simulink model "SimulationOfFuruta"  (R2017a)
settings: Solver=ode4  StartTime=0.0  StopTime=20  RelTol=1e-3  EnableMultiTasking=on
settings Model: Creator=marce  LastModifiedBy=felip
settings DataIOCC: LimitDataPoints=on  SaveFormat=Array
settings OptimizationCC: LifeSpan=inf
settings DebuggingCC: SFUnexpectedBacktrackingDiag=warning  SFNoUnconditionalDefaultTransitionDiag=warning  SFExecutionAtInitializationDiag=none
settings HardwareCC: ProdBitPerPointer=32  ProdBitPerSizeT=32  ProdBitPerPtrDiffT=32  ProdLargestAtomicFloat=None  ProdIntDivRoundTo=Undefined  ProdEndianess=Unspecified  ProdWordSize=32  ProdHWDeviceType=32-bit Generic
settings ModelReferenceCC: PropagateSignalLabelsOutOfModel=off
settings GRTTargetCC: TargetLangStandard=C89/C90 (ANSI)  GeneratePreprocessorConditionals=Disable all
settings ConfigComp: CovMetricSettings=dw  CovHtmlReporting=on  CovSaveCumulativeToWorkspaceVar=on  CovSaveSingleToWorkspaceVar=on  CovExternalEMLEnable=off

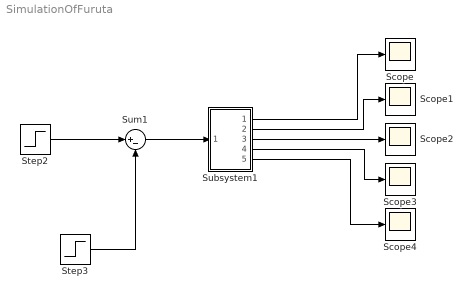
== system SimulationOfFuruta ==
  Scope{,1..4} (5 alike) : Scope
  Step2 : Step  SampleTime=0
  Step3 : Step  SampleTime=0
  Subsystem1 : Subsystem
  Sum1 : Sum  Inputs=|+-
  wires:
  Subsystem1/4(Out4) -> Scope3/1
  Subsystem1/3(Out3) -> Scope2/1
  Subsystem1/5(Out5) -> Scope4/1
  Subsystem1/2(Out2) -> Scope1/1
  Subsystem1/1(Out1) -> Scope/1
  Step3/1 -> Sum1/2
  Step2/1 -> Sum1/1
  Sum1/1 -> Subsystem1/1(In1)

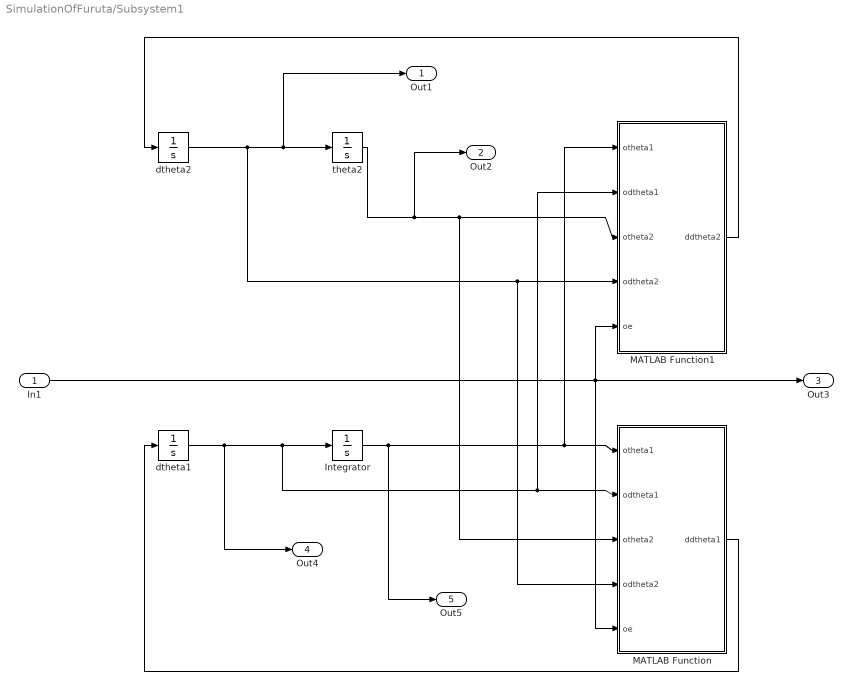
== system SimulationOfFuruta/Subsystem1 ==
  In1 : Inport
  Integrator : Integrator
  MATLAB Function : MATLAB Function  TreatAsAtomicUnit=on
  MATLAB Function1 : MATLAB Function  TreatAsAtomicUnit=on
  dtheta1 : Integrator
  dtheta2 : Integrator
  theta2 : Integrator
  Out1 : Outport
  Out2 : Outport  Port=2
  Out3 : Outport  Port=3
  Out4 : Outport  Port=4
  Out5 : Outport  Port=5
  wires:
  dtheta2/1 -> MATLAB Function/4(odtheta2), MATLAB Function1/4(odtheta2), Out1/1, theta2/1
  dtheta1/1 -> Out4/1, MATLAB Function1/2(odtheta1), MATLAB Function/2(odtheta1), Integrator/1
  Integrator/1 -> Out5/1, MATLAB Function/1(otheta1), MATLAB Function1/1(otheta1)
  MATLAB Function/1(ddtheta1) -> dtheta1/1
  In1/1 -> MATLAB Function/5(oe), Out3/1, MATLAB Function1/5(oe)
  theta2/1 -> Out2/1, MATLAB Function/3(otheta2), MATLAB Function1/3(otheta2)
  MATLAB Function1/1(ddtheta2) -> dtheta2/1

== matlab function SimulationOfFuruta/Subsystem1/MATLAB Function ==
  data: otheta1 input; odtheta1 input; ddtheta1 output; otheta2 input; odtheta2 input; oe input
function ddtheta1 = fcn1(otheta1,odtheta1,otheta2,odtheta2,oe)

ddtheta1 = zeros(1,1);  
coder.extrinsic('syms')
syms theta1 dtheta1 theta2 dtheta2 e;
Func1=symfun((273383219505647715290264984433600000000*dtheta1 - 198062144703003418648387563281250000000*e - 416088040453654448350580039910539919360000*sin(2*theta2) + 13560500260173729040508156862701670236160*dtheta2^2*sin(theta2) - 13439683643334208660240022593773670236160*dtheta1^2*(sin(theta2) - sin(theta2)^3) + 16266042072052499191574494429931640625*dtheta2*cos(theta2) + 9142176042555954133369991857325960331264*dtheta1*dtheta2*sin(2*theta2))/(696932042335584256*(41721610581794358547444*cos(theta2)^2 - 229801380526943752815105)),[theta1 dtheta1 theta2 dtheta2 e])
ddtheta1=vpa(subs(Func1,[theta1 dtheta1 theta2 dtheta2 e],[odtheta1,otheta1,odtheta2,otheta2,oe]));

== matlab function SimulationOfFuruta/Subsystem1/MATLAB Function1 ==
  data: otheta1 input; odtheta1 input; ddtheta2 output; otheta2 input; odtheta2 input; oe input
function ddtheta2 = fcn2(otheta1,odtheta1,otheta2,odtheta2,oe)

ddtheta2 = zeros(1,1);  
coder.extrinsic('syms')
syms theta1 dtheta1 theta2 dtheta2 e;
Func2=symfun((1536877429000564048815928821109619140625*dtheta2 - 78627156504041188505523135421261472071680000*sin(theta2) - 634916175454785429479332065228843667947520*dtheta1^2*sin(2*theta2) + 79739804918975647357573983605853100441600*dtheta2^2*sin(2*theta2) + 3215150499355185931248636722272000000000*dtheta1*cos(theta2) - 2329329519919803072008927828125000000000*e*cos(theta2) - 4488271131060137965939268641213019848704000*sin(theta2)*(sin(theta2)^2 - 1) - 87729518696337784553411358347656250000*dtheta2*cos(theta2)^2 + 215034938293347338563840361500378723778560*dtheta1*dtheta2*(sin(theta2) - sin(theta2)^3) + 72485794161724834273391887682518082650112*dtheta1^2*cos(theta2)^3*sin(theta2))/(5575456338684674048*(41721610581794358547444*cos(theta2)^2 - 229801380526943752815105)),[theta1 dtheta1 theta2 dtheta2 e])
ddtheta2 = vpa(subs(Func2,[theta1 dtheta1 theta2 dtheta2 e],[odtheta1,otheta1,odtheta2,otheta2,oe]));
